simulink model "ControladorLuces"  (R2022b)
settings: Solver=VariableStepAuto  StartTime=0.0  StopTime=10.0  RelTol=1e-3
libraries: simulink x6
settings Model: Creator=laura  LastModifiedBy=laura

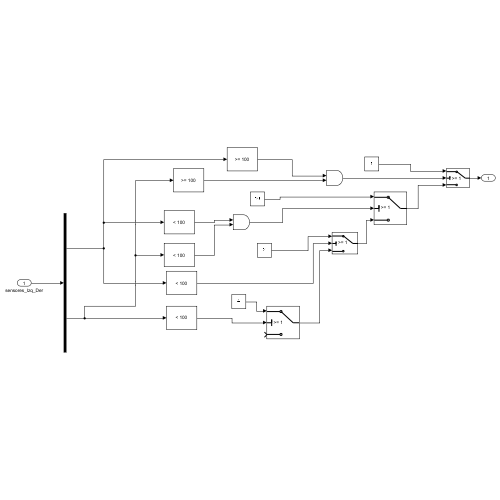
[thumbnail: Simulink's stored preview of the top-level diagram]
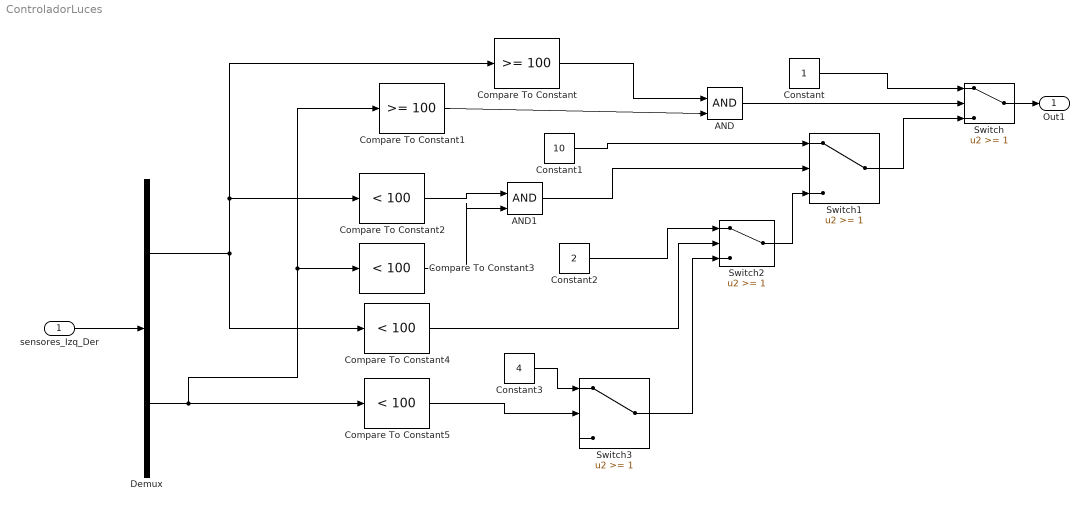
== system ControladorLuces ==
  sensores_Izq_Der : Inport
  AND : Logic  IconShape=distinctive  AllPortsSameDT=off  OutDataTypeStr=boolean
  AND1 : Logic  IconShape=distinctive  AllPortsSameDT=off  OutDataTypeStr=boolean
  Compare To Constant : simulink/Logic and Bit Operations/Compare To Constant  relop=>=  const=100  OutDataTypeStr=boolean
  Compare To Constant1 : simulink/Logic and Bit Operations/Compare To Constant  relop=>=  const=100  OutDataTypeStr=boolean
  Compare To Constant{2..5} (4 alike) : simulink/Logic and Bit Operations/Compare To Constant  relop=<  const=100  OutDataTypeStr=boolean
  Constant : Constant
  Constant1 : Constant  Value=10
  Constant2 : Constant  Value=2
  Constant3 : Constant  Value=4
  Demux : Demux  Outputs=2
  Switch{,1..3} (4 alike) : Switch  Threshold=1  SaturateOnIntegerOverflow=off  InputSameDT=off
  Out1 : Outport
  wires:
  Compare To Constant2/1 -> AND1/1
  Switch/1 -> Out1/1
  Compare To Constant5/1 -> Switch3/2
  Switch3/1 -> Switch2/3
  Compare To Constant4/1 -> Switch2/2
  Constant1/1 -> Switch1/1
  Compare To Constant1/1 -> AND/2
  AND1/1 -> Switch1/2
  Constant2/1 -> Switch2/1
  Compare To Constant3/1 -> AND1/2
  Demux/2 -> Compare To Constant5/1, Compare To Constant3/1, Compare To Constant1/1
  Constant3/1 -> Switch3/1
  Compare To Constant/1 -> AND/1
  Constant/1 -> Switch/1
  Demux/1 -> Compare To Constant/1, Compare To Constant2/1, Compare To Constant4/1
  sensores_Izq_Der/1 -> Demux/1
  Switch2/1 -> Switch1/3
  Switch1/1 -> Switch/3
  AND/1 -> Switch/2
